simulink model "Benchmark_IEEE_standardn4"  (R2018a)
settings: Solver=ode45  StartTime=0.0  StopTime=200  FixedStep=1e-4  RelTol=1e-5  EnableMultiTasking=on
undefined symbols (not defined in the file): a, Aex, b, Bex, D, delta0, dVref, Ed_dash0, Edc_dash0, Efd0, Efdmax, Efdmax_dc, Efdmin, Efdmin_dc, Eq_dash0, j, Ka, KA, Kad, kc, Kd, Ke, Kf, Ki, Kp, Ks, M, MM, P18cor2, P50cor2, Psi1d0, Psi2q0, Sm0, T11, T12, T21, T22, T31, T32, Ta, Tc, Td, Td0d, Td0dd, Te, Tf, theta, Tm0, Tq0d, Tq0dd, Tr, Tw, V, v1, V18cor, V2, V50cor, V_Ka0, V_Ki0, Vg ... (+15)
settings Model: Creator=aks11  LastModifiedBy=sanam
settings DataIOCC: SaveFormat=StructureWithTime  SignalLoggingSaveFormat=ModelDataLogs  SaveOutput=off  SaveState=on  SignalLogging=off  DSMLogging=off
settings OptimizationCC: BlockReduction=off  DefaultParameterBehavior=Inlined  BufferReuse=off  ExpressionDepthLimit=2147483647  LifeSpan=inf  SimCompilerOptimization=on
settings DebuggingCC: AlgebraicLoopMsg=none  UnderspecifiedInitializationDetection=Classic  MergeDetectMultiDrivingBlocksExec=none  FcnCallInpInsideContextMsg=warning  UnconnectedInputMsg=none  UnconnectedOutputMsg=none  UnconnectedLineMsg=none  StateNameClashWarn=warning  SFUnexpectedBacktrackingDiag=warning  SFNoUnconditionalDefaultTransitionDiag=warning  SFExecutionAtInitializationDiag=none
settings HardwareCC: ProdBitPerPointer=32  ProdBitPerSizeT=32  ProdBitPerPtrDiffT=32  ProdLargestAtomicFloat=None  ProdIntDivRoundTo=Undefined  ProdEndianess=Unspecified  ProdWordSize=32  ProdHWDeviceType=32-bit Generic
settings ModelReferenceCC: PropagateSignalLabelsOutOfModel=off
settings CodeAppCC: StateflowObjectComments=on
settings GRTTargetCC: TargetLangStandard=C89/C90 (ANSI)  GeneratePreprocessorConditionals=Disable all  CombineOutputUpdateFcns=off  GRTInterface=on
settings ConfigComp: CovMetricSettings=dw  CovHtmlReporting=on  CovSaveCumulativeToWorkspaceVar=on  CovSaveSingleToWorkspaceVar=on  CovExternalEMLEnable=off

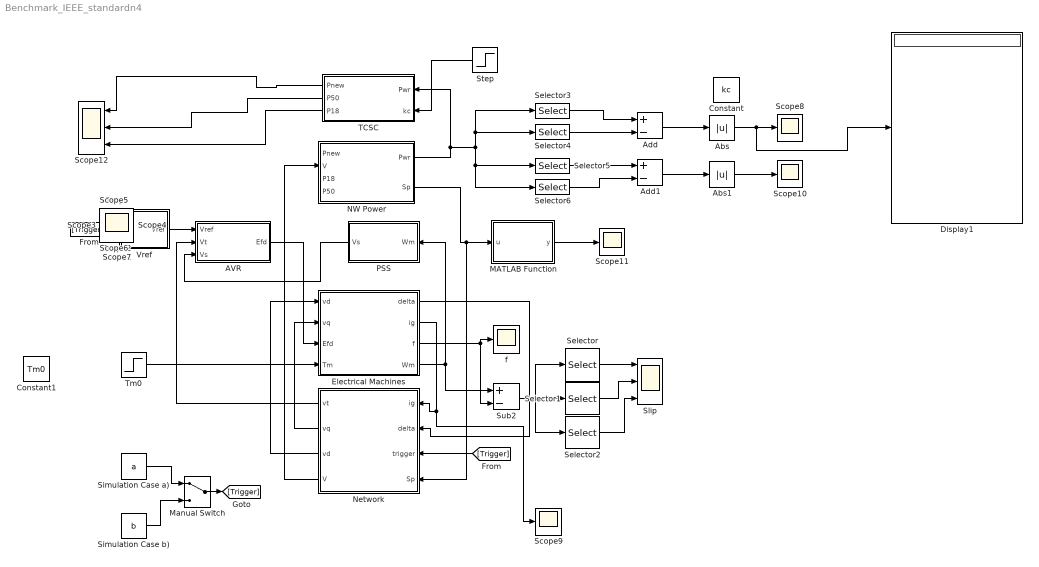
== system Benchmark_IEEE_standardn4 ==
  AVR : Subsystem
  Abs : Abs
  Abs1 : Abs
  Add : Sum  Inputs=+-
  Add1 : Sum  Inputs=+-
  Constant : Constant  Value=kc
  Constant1 : Constant  Value=Tm0
  Display1 : Display
  Electrical Machines : Subsystem
  MATLAB Function : MATLAB Function  TreatAsAtomicUnit=on
  Manual Switch : ManualSwitch
  NW Power : Subsystem
  Network : Subsystem
  PSS : Subsystem
  Scope{,1..11} (12 alike) : Scope
  Scope12 : Scope  NumInputPorts=3
  Selector : Selector  IndexOptions=Index vector (dialog)  Indices=4  OutputSizes=1
  Selector1 : Selector  IndexOptions=Index vector (dialog)  Indices=9  OutputSizes=1
  Selector2 : Selector  IndexOptions=Index vector (dialog)  Indices=15  OutputSizes=1
  Selector3 : Selector  IndexOptions=Index vector (dialog)  Indices=13  OutputSizes=1
  Selector4 : Selector  IndexOptions=Index vector (dialog)  Indices=17  OutputSizes=1
  Selector5 : Selector  IndexOptions=Index vector (dialog)  Indices=16  OutputSizes=1
  Selector6 : Selector  IndexOptions=Index vector (dialog)  Indices=18  OutputSizes=1
  Simulation Case a) : Constant  Value=a
  Simulation Case b) : Constant  Value=b
  Slip : Scope  NumInputPorts=3
  Step : Step  Time=0  After=0.5  SampleTime=0
  Sub2 : Sum  Inputs=+-
  TCSC : Subsystem
  Tm0 : Step  Time=0  Before=Tm0  After=Tm0  SampleTime=0
  Vref : Subsystem
  f : Scope
  wires:
  Electrical Machines/2(ig) -> Scope9/1, Network/1(ig)
  Network/1(vt) -> AVR/2(Vt)
  Network/2(vq) -> Electrical Machines/2(vq)
  Network/3(vd) -> Electrical Machines/1(vd)
  Tm0/1 -> Electrical Machines/4(Tm)
  PSS/1(Vs) -> AVR/3(Vs)
  AVR/1(Efd) -> Electrical Machines/3("Efd ")
  Selector/1 -> Slip/1
  Electrical Machines/3(f) -> f/1, Sub2/2
  Electrical Machines/4(Wm) -> Sub2/1, PSS/1(Wm)
  Electrical Machines/1(delta) -> Network/2(delta)
  Sub2/1 -> Selector2/1, Selector/1, Selector1/1
  Vref/1(Vref) -> AVR/1(Vref)
  Simulation Case a)/1 -> Manual Switch/1
  Simulation Case b)/1 -> Manual Switch/2
  Manual Switch/1 -> [Trigger]
  [Trigger] -> Vref/1(trigger)
  [Trigger] -> Network/3(trigger)
  Selector1/1 -> Slip/2
  Selector2/1 -> Slip/3
  NW Power/1(Pwr) -> Selector3/1, Selector4/1, Selector6/1, Selector5/1, TCSC/1(Pwr)
  TCSC/1(Pnew) -> Scope12/1
  TCSC/2(P50) -> Scope12/2
  TCSC/3(P18) -> Scope12/3
  Selector3/1 -> Add/1
  Selector4/1 -> Add/2
  Selector5/1 -> Add1/1
  Selector6/1 -> Add1/2
  Add/1 -> Abs/1
  Add1/1 -> Abs1/1
  Abs/1 -> Display1/1, Scope8/1
  Abs1/1 -> Scope10/1
  NW Power/2(Sp) -> Network/4(Sp), MATLAB Function/1(u)
  MATLAB Function/1(y) -> Scope11/1
  Network/4(V) -> NW Power/2(V)
  Step/1 -> TCSC/2(kc)

== system Benchmark_IEEE_standardn4/AVR ==
  Vref : Inport
  Vt : Inport  Port=2
  Vs : Inport  Port=3
  AVR (DC4B) : Subsystem
  AVR (ST1A) : Subsystem
  Manual : Subsystem
  Sum7 : Sum  Inputs=+++
  Efd : Outport
  wires:
  Sum7/1 -> Efd/1
  AVR (DC4B)/1(Efd) -> Sum7/2
  AVR (ST1A)/1(Efd) -> Sum7/1
  Vref/1 -> Manual/1(Vref), AVR (DC4B)/1(Vref), AVR (ST1A)/1(Vref)
  Vt/1 -> AVR (DC4B)/2(Vt), AVR (ST1A)/2(Vt)
  Vs/1 -> AVR (DC4B)/3(Vs), AVR (ST1A)/3(Vs)
  Manual/1(Efd3) -> Sum7/3

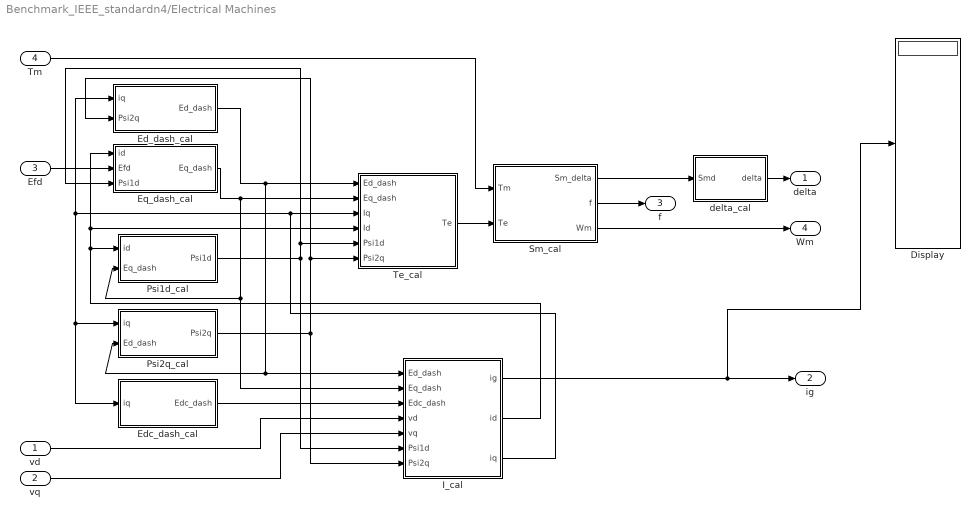
== system Benchmark_IEEE_standardn4/Electrical Machines ==
  vd : Inport
  vq : Inport  Port=2
  "Efd " : Inport  Port=3
  Tm : Inport  Port=4
  Display : Display
  Ed_dash_cal : Subsystem
  Edc_dash_cal : Subsystem
  Eq_dash_cal : Subsystem
  I_cal : Subsystem
  Psi1d_cal : Subsystem
  Psi2q_cal : Subsystem
  Sm_cal : Subsystem
  Te_cal : Subsystem
  delta_cal : Subsystem
  delta : Outport
  ig : Outport  Port=2
  f : Outport  Port=3
  Wm : Outport  Port=4
  wires:
  Ed_dash_cal/1(Ed_dash) -> Te_cal/1(Ed_dash), I_cal/1(Ed_dash), Psi2q_cal/2(Ed_dash)
  Eq_dash_cal/1(Eq_dash) -> Te_cal/2(Eq_dash), I_cal/2(Eq_dash), Psi1d_cal/2(Eq_dash)
  "Efd "/1 -> Eq_dash_cal/2(Efd)
  Edc_dash_cal/1(Edc_dash) -> I_cal/3(Edc_dash)
  vd/1 -> I_cal/4(vd)
  vq/1 -> I_cal/5(vq)
  I_cal/3(iq) -> Te_cal/3(Iq), Ed_dash_cal/1(iq), Edc_dash_cal/1(iq), Psi2q_cal/1(iq)
  I_cal/1(ig) -> Display/1, ig/1
  I_cal/2(id) -> Eq_dash_cal/1(id), Te_cal/4(Id), Psi1d_cal/1(id)
  Psi2q_cal/1(Psi2q) -> Te_cal/6(Psi2q), Ed_dash_cal/2(Psi2q), I_cal/7(Psi2q)
  Psi1d_cal/1(Psi1d) -> Te_cal/5(Psi1d), Eq_dash_cal/3(Psi1d), I_cal/6(Psi1d)
  Sm_cal/2(f) -> f/1
  Sm_cal/1(Sm_delta) -> delta_cal/1(Smd)
  delta_cal/1(delta) -> delta/1
  Sm_cal/3(Wm) -> Wm/1
  Te_cal/1(Te) -> Sm_cal/2(Te)
  Tm/1 -> Sm_cal/1(Tm)

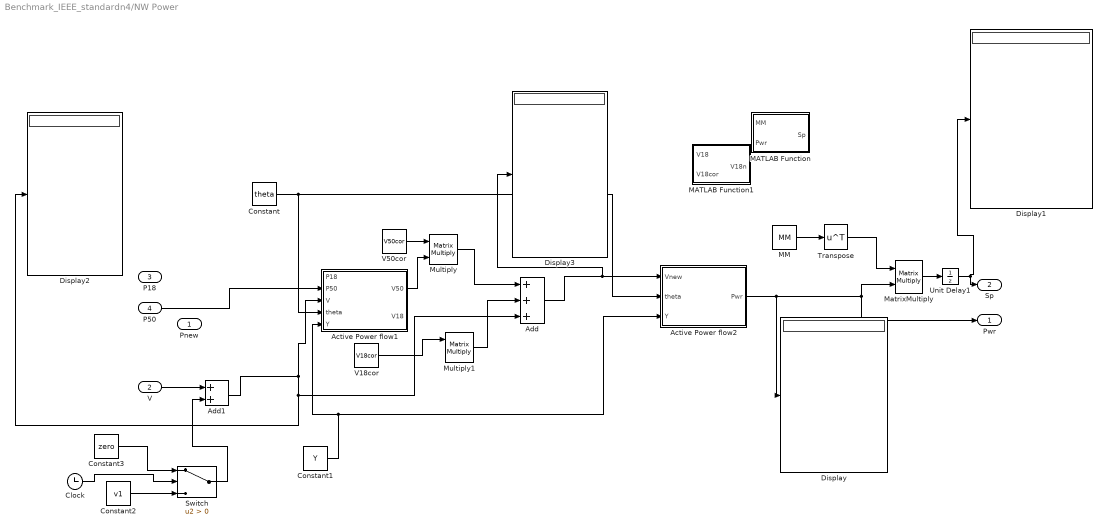
== system Benchmark_IEEE_standardn4/NW Power ==
  Pnew : Inport
  V : Inport  Port=2
  P18 : Inport  Port=3
  P50 : Inport  Port=4
  Active Power flow1 : MATLAB Function  TreatAsAtomicUnit=on
  Active Power flow2 : MATLAB Function  TreatAsAtomicUnit=on
  Add : Sum  Inputs=3
  Add1 : Sum
  Clock : Clock
  Constant : Constant  Value=theta
  Constant1 : Constant  Value=Y
  Constant2 : Constant  Value=v1
  Constant3 : Constant  Value=zero
  Display{,1..3} (4 alike) : Display
  MATLAB Function : MATLAB Function  TreatAsAtomicUnit=on
  MATLAB Function1 : MATLAB Function  TreatAsAtomicUnit=on
  MM : Constant  Value=MM
  MatrixMultiply : Product  Multiplication=Matrix(*)
  Multiply : Product  Multiplication=Matrix(*)
  Multiply1 : Product  Multiplication=Matrix(*)
  Switch : Switch  Criteria=u2 > Threshold
  Transpose : Math  Operator=transpose  SaturateOnIntegerOverflow=on
  Unit Delay1 : UnitDelay  SampleTime=-1
  V18cor : Constant  Value=V18cor
  V50cor : Constant  Value=V50cor
  Pwr : Outport
  Sp : Outport  Port=2
  wires:
  Constant1/1 -> Active Power flow1/5(Y), Active Power flow2/3(Y)
  Constant/1 -> Active Power flow1/4(theta), Active Power flow2/2(theta)
  V50cor/1 -> Multiply/1
  Active Power flow1/1(V50) -> Multiply/2
  Multiply/1 -> Add/1
  Active Power flow2/1(Pwr) -> Display/1, MatrixMultiply/2, Pwr/1
  MM/1 -> Transpose/1
  Multiply1/1 -> Add/2
  Unit Delay1/1 -> Display1/1, Sp/1
  MatrixMultiply/1 -> Unit Delay1/1
  V18cor/1 -> Multiply1/1
  Add/1 -> Display3/1, Active Power flow2/1(Vnew)
  Transpose/1 -> MatrixMultiply/1
  Add1/1 -> Display2/1, Add/3, Active Power flow1/3(V)
  V/1 -> Add1/1
  Constant2/1 -> Switch/3
  Clock/1 -> Switch/2
  Constant3/1 -> Switch/1
  Switch/1 -> Add1/2
  P50/1 -> Active Power flow1/2(P50)

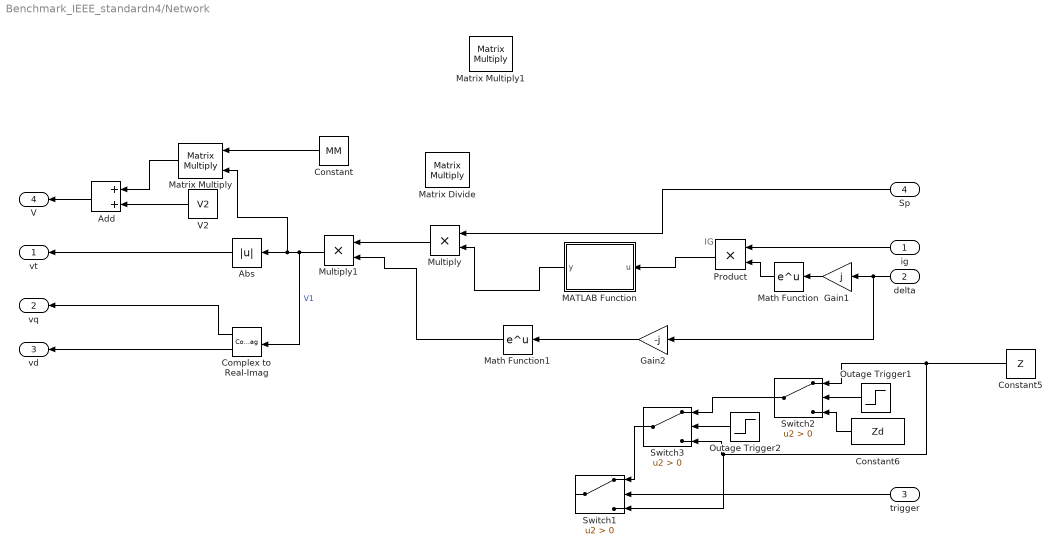
== system Benchmark_IEEE_standardn4/Network ==
  note: IG
  ig : Inport
  delta : Inport  Port=2
  trigger : Inport  Port=3
  Sp : Inport  Port=4
  Abs : Abs
  Add : Sum
  Complex to Real-Imag : ComplexToRealImag
  Constant : Constant  Value=MM
  Constant5 : Constant  Value=Z
  Constant6 : Constant  Value=Zd
  Gain1 : Gain  Gain=j
  Gain2 : Gain  Gain=-j
  MATLAB Function : MATLAB Function  TreatAsAtomicUnit=on
  Math Function : Math  SaturateOnIntegerOverflow=on
  Math Function1 : Math  SaturateOnIntegerOverflow=on
  Matrix Divide : Product  Inputs=**  Multiplication=Matrix(*)
  Matrix Multiply : Product  Multiplication=Matrix(*)
  Matrix Multiply1 : Product  Multiplication=Matrix(*)
  Multiply : Product
  Multiply1 : Product
  Outage Trigger1 : Step  Before=1  After=0  SampleTime=0
  Outage Trigger2 : Step  Time=11  Before=1  After=0  SampleTime=0
  Product : Product  RndMeth=Zero
  Switch1 : Switch  Criteria=u2 > Threshold
  Switch2 : Switch  Criteria=u2 > Threshold
  Switch3 : Switch  Criteria=u2 > Threshold
  V2 : Constant  Value=V2
  vt : Outport
  vq : Outport  Port=2
  vd : Outport  Port=3
  V : Outport  Port=4
  wires:
  Math Function/1 -> Product/2
  Math Function1/1 -> Multiply1/2
  Gain2/1 -> Math Function1/1
  Gain1/1 -> Math Function/1
  Abs/1 -> vt/1
  Complex to Real-Imag/1 -> vq/1
  ig/1 -> Product/1
  Multiply1/1 -> Complex to Real-Imag/1, Matrix Multiply/2, Abs/1  "V1"
  Multiply/1 -> Multiply1/1
  delta/1 -> Gain2/1, Gain1/1
  Outage Trigger1/1 -> Switch2/2
  Constant6/1 -> Switch2/3
  Complex to Real-Imag/2 -> vd/1
  Outage Trigger2/1 -> Switch3/2
  Switch2/1 -> Switch3/1
  Switch3/1 -> Switch1/1
  trigger/1 -> Switch1/2
  Constant5/1 -> Switch1/3, Switch3/3, Switch2/1
  Product/1 -> MATLAB Function/1(u)
  Sp/1 -> Multiply/1
  Constant/1 -> Matrix Multiply/1
  Matrix Multiply/1 -> Add/1
  V2/1 -> Add/2
  Add/1 -> V/1
  MATLAB Function/1(y) -> Multiply/2

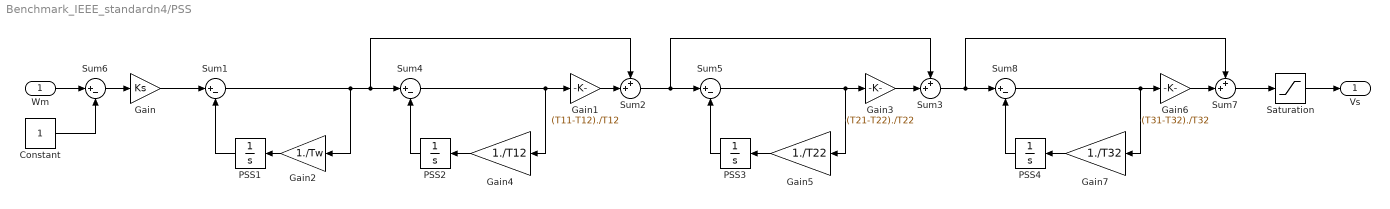
== system Benchmark_IEEE_standardn4/PSS ==
  Wm : Inport
  Constant : Constant
  Gain : Gain  Gain=Ks
  Gain1 : Gain  Gain=(T11-T12)./T12
  Gain2 : Gain  Gain=1./Tw
  Gain3 : Gain  Gain=(T21-T22)./T22
  Gain4 : Gain  Gain=1./T12
  Gain5 : Gain  Gain=1./T22
  Gain6 : Gain  Gain=(T31-T32)./T32
  Gain7 : Gain  Gain=1./T32
  PSS{1..4} (4 alike) : Integrator  UpperSaturationLimit=Efdmax  LowerSaturationLimit=Efdmin
  Saturation : Saturate  UpperLimit=Vs_max  LowerLimit=Vs_min
  Sum{1,4..6,8} (5 alike) : Sum  Inputs=|+-
  Sum2 : Sum  Inputs=++|
  Sum3 : Sum  Inputs=++|
  Sum7 : Sum  Inputs=++|
  Vs : Outport
  wires:
  Gain/1 -> Sum1/1
  Saturation/1 -> Vs/1
  Sum1/1 -> Gain2/1, Sum4/1, Sum2/1
  PSS1/1 -> Sum1/2
  Gain2/1 -> PSS1/1
  Sum4/1 -> Gain4/1, Gain1/1
  PSS2/1 -> Sum4/2
  Gain4/1 -> PSS2/1
  Gain1/1 -> Sum2/2
  Sum2/1 -> Sum3/1, Sum5/1
  Sum5/1 -> Gain3/1, Gain5/1
  PSS3/1 -> Sum5/2
  Gain5/1 -> PSS3/1
  Gain3/1 -> Sum3/2
  Wm/1 -> Sum6/1
  Sum6/1 -> Gain/1
  Constant/1 -> Sum6/2
  Sum7/1 -> Saturation/1
  Sum3/1 -> Sum7/1, Sum8/1
  Sum8/1 -> Gain6/1, Gain7/1
  PSS4/1 -> Sum8/2
  Gain7/1 -> PSS4/1
  Gain6/1 -> Sum7/2

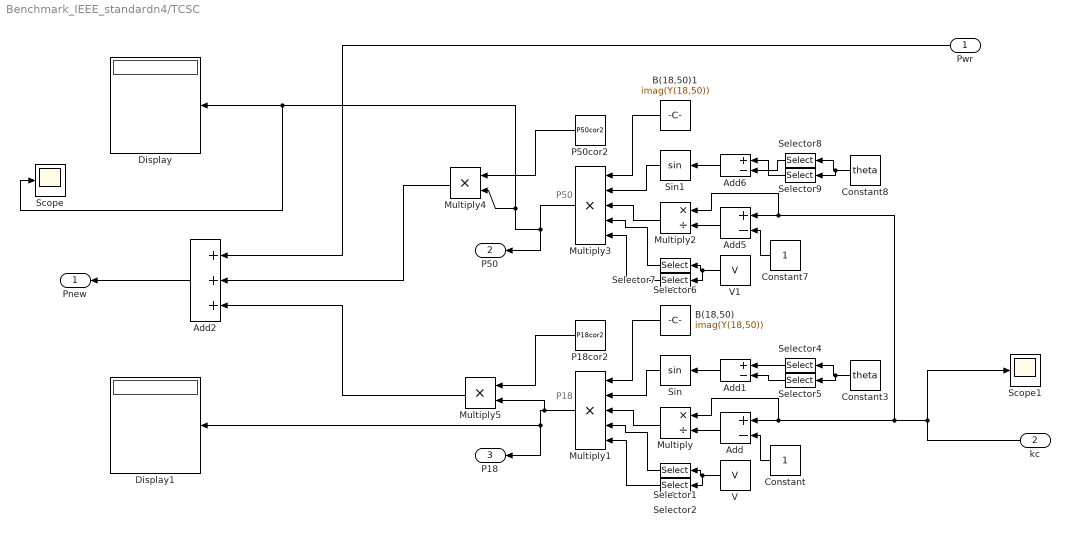
== system Benchmark_IEEE_standardn4/TCSC ==
  note: P18
  note: P50
  Pwr : Inport
  kc : Inport  Port=2
  Add{,1,5..6} (4 alike) : Sum  Inputs=+-
  Add2 : Sum  Inputs=3
  B(18,50) : Constant  Value=imag(Y(18,50))
  B(18,50)1 : Constant  Value=imag(Y(18,50))
  Constant : Constant
  Constant3 : Constant  Value=theta
  Constant7 : Constant
  Constant8 : Constant  Value=theta
  Display : Display
  Display1 : Display
  Multiply : Product  Inputs=*/
  Multiply1 : Product  Inputs=*****
  Multiply2 : Product  Inputs=*/
  Multiply3 : Product  Inputs=*****
  Multiply4 : Product
  Multiply5 : Product
  P18cor2 : Constant  Value=P18cor2
  P50cor2 : Constant  Value=P50cor2
  Scope : Scope
  Scope1 : Scope
  Selector{1,4,6,8} (4 alike) : Selector  IndexOptions=Index vector (dialog)  Indices=18  OutputSizes=1
  Selector{2,5,7,9} (4 alike) : Selector  IndexOptions=Index vector (dialog)  Indices=50  OutputSizes=1
  Sin : Trigonometry
  Sin1 : Trigonometry
  V : Constant  Value=V
  V1 : Constant  Value=V
  Pnew : Outport
  P50 : Outport  Port=2
  P18 : Outport  Port=3
  wires:
  Sin/1 -> Multiply1/2
  B(18,50)/1 -> Multiply1/1
  Multiply2/1 -> Multiply3/3
  Constant7/1 -> Add5/2
  V/1 -> Selector2/1, Selector1/1
  Sin1/1 -> Multiply3/2
  kc/1 -> Scope1/1, Multiply2/1, Add5/1, Multiply/1, Add/1
  Selector2/1 -> Multiply1/5
  V1/1 -> Selector7/1, Selector6/1
  Add/1 -> Multiply/2
  B(18,50)1/1 -> Multiply3/1
  Multiply/1 -> Multiply1/3
  Constant/1 -> Add/2
  Selector7/1 -> Multiply3/5
  Constant8/1 -> Selector9/1, Selector8/1
  Selector6/1 -> Multiply3/4
  Constant3/1 -> Selector5/1, Selector4/1
  Add6/1 -> Sin1/1
  Selector1/1 -> Multiply1/4
  Add1/1 -> Sin/1
  Selector4/1 -> Add1/1
  Selector5/1 -> Add1/2
  Add5/1 -> Multiply2/2
  Selector9/1 -> Add6/1
  Selector8/1 -> Add6/2
  P50cor2/1 -> Multiply4/1
  P18cor2/1 -> Multiply5/1
  Pwr/1 -> Add2/1
  Multiply4/1 -> Add2/2
  Multiply5/1 -> Add2/3
  Multiply1/1 -> Multiply5/2, Display1/1, P18/1
  Multiply3/1 -> Multiply4/2, Scope/1, Display/1, P50/1
  Add2/1 -> Pnew/1

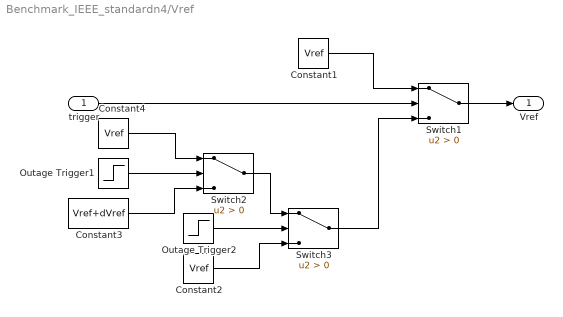
== system Benchmark_IEEE_standardn4/Vref ==
  trigger : Inport
  Constant1 : Constant  Value=Vref
  Constant2 : Constant  Value=Vref
  Constant3 : Constant  Value=Vref+dVref
  Constant4 : Constant  Value=Vref
  Outage Trigger1 : Step  Before=1  After=0  SampleTime=0
  Outage Trigger2 : Step  Time=11  Before=1  After=0  SampleTime=0
  Switch1 : Switch  Criteria=u2 > Threshold
  Switch2 : Switch  Criteria=u2 > Threshold
  Switch3 : Switch  Criteria=u2 > Threshold
  Vref : Outport
  wires:
  Constant1/1 -> Switch1/1
  Constant2/1 -> Switch3/3
  Outage Trigger2/1 -> Switch3/2
  Switch3/1 -> Switch1/3
  Switch1/1 -> Vref/1
  Constant3/1 -> Switch2/3
  Outage Trigger1/1 -> Switch2/2
  Switch2/1 -> Switch3/1
  Constant4/1 -> Switch2/1
  trigger/1 -> Switch1/2

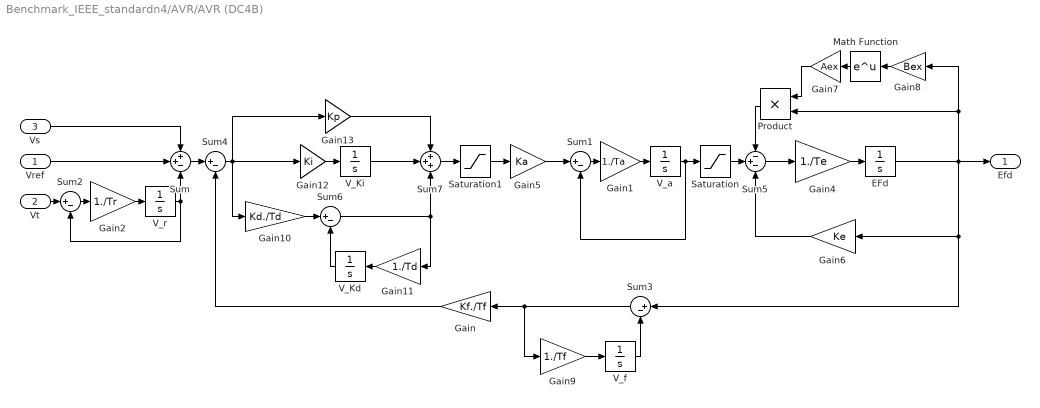
== system Benchmark_IEEE_standardn4/AVR/AVR (DC4B) ==
  Vref : Inport
  Vt : Inport  Port=2
  Vs : Inport  Port=3
  EFd : Integrator  InitialCondition=Efd0.*Kad  UpperSaturationLimit=Efdmax_dc  LowerSaturationLimit=Efdmin_dc
  Gain : Gain  Gain=Kf./Tf
  Gain1 : Gain  Gain=1./Ta
  Gain10 : Gain  Gain=Kd./Td
  Gain11 : Gain  Gain=1./Td
  Gain12 : Gain  Gain=Ki
  Gain13 : Gain  Gain=Kp
  Gain2 : Gain  Gain=1./Tr
  Gain4 : Gain  Gain=1./Te
  Gain5 : Gain  Gain=Ka
  Gain6 : Gain  Gain=Ke
  Gain7 : Gain  Gain=Aex
  Gain8 : Gain  Gain=Bex
  Gain9 : Gain  Gain=1./Tf
  Math Function : Math  SaturateOnIntegerOverflow=on
  Product : Product  RndMeth=Zero
  Saturation : Saturate  UpperLimit=Efdmax_dc  LowerLimit=Efdmin_dc
  Saturation1 : Saturate  UpperLimit=Efdmax_dc./Ka  LowerLimit=Efdmin_dc./Ka
  Sum : Sum  Inputs=++-
  Sum{1..4,6} (5 alike) : Sum  Inputs=|+-
  Sum5 : Sum  Inputs=-+-
  Sum7 : Sum  Inputs=+++
  V_Kd : Integrator  UpperSaturationLimit=Efdmax  LowerSaturationLimit=Efdmin
  V_Ki : Integrator  InitialCondition=V_Ki0  UpperSaturationLimit=Efdmax_dc  LowerSaturationLimit=Efdmin_dc
  V_a : Integrator  InitialCondition=V_Ka0  UpperSaturationLimit=Efdmax  LowerSaturationLimit=Efdmin
  V_f : Integrator  InitialCondition=Efd0.*Kad  UpperSaturationLimit=Efdmax  LowerSaturationLimit=Efdmin
  V_r : Integrator  InitialCondition=Vg  UpperSaturationLimit=Efdmax  LowerSaturationLimit=Efdmin
  Efd : Outport
  wires:
  Gain8/1 -> Math Function/1
  Math Function/1 -> Gain7/1
  Sum1/1 -> Gain1/1
  Gain1/1 -> V_a/1
  V_a/1 -> Sum1/2, Saturation/1
  Gain5/1 -> Sum1/1
  Sum5/1 -> Gain4/1
  Gain4/1 -> EFd/1
  Sum2/1 -> Gain2/1
  Gain2/1 -> V_r/1
  V_r/1 -> Sum2/2, Sum/3
  Vref/1 -> Sum/2
  Vt/1 -> Sum2/1
  Product/1 -> Sum5/1
  Gain6/1 -> Sum5/3
  Gain7/1 -> Product/1
  Saturation/1 -> Sum5/2
  EFd/1 -> Product/2, Gain8/1, Efd/1, Sum3/1, Gain6/1
  Gain9/1 -> V_f/1
  Sum3/1 -> Gain/1, Gain9/1
  Sum/1 -> Sum4/1
  V_Kd/1 -> Sum6/2
  Gain11/1 -> V_Kd/1
  Gain10/1 -> Sum6/1
  Sum6/1 -> Sum7/3, Gain11/1
  Gain12/1 -> V_Ki/1
  V_Ki/1 -> Sum7/2
  Gain13/1 -> Sum7/1
  Sum7/1 -> Saturation1/1
  Sum4/1 -> Gain13/1, Gain12/1, Gain10/1
  Saturation1/1 -> Gain5/1
  Vs/1 -> Sum/1
  V_f/1 -> Sum3/2
  Gain/1 -> Sum4/2

== system Benchmark_IEEE_standardn4/AVR/AVR (ST1A) ==
  Vref : Inport
  Vt : Inport  Port=2
  Vs : Inport  Port=3
  EFdd2 : Integrator  InitialCondition=Vg  UpperSaturationLimit=Efdmax  LowerSaturationLimit=Efdmin
  Gain2 : Gain  Gain=1./Tr
  Gain5 : Gain  Gain=KA
  Saturation : Saturate  UpperLimit=Efdmax  LowerLimit=Efdmin
  Sum : Sum  Inputs=++-
  Sum2 : Sum  Inputs=|+-
  Efd : Outport
  wires:
  Saturation/1 -> Efd/1
  Gain5/1 -> Saturation/1
  Sum2/1 -> Gain2/1
  Gain2/1 -> EFdd2/1
  EFdd2/1 -> Sum2/2, Sum/3
  Vref/1 -> Sum/2
  Vs/1 -> Sum/1
  Vt/1 -> Sum2/1
  Sum/1 -> Gain5/1

== system Benchmark_IEEE_standardn4/AVR/Manual ==
  Vref : Inport
  Gain9 : Gain  Gain=Vref_Manual
  Efd3 : Outport
  wires:
  Vref/1 -> Gain9/1
  Gain9/1 -> Efd3/1

== system Benchmark_IEEE_standardn4/Electrical Machines/Ed_dash_cal ==
  iq : Inport
  Psi2q : Inport  Port=2
  Add2 : Sum  Inputs=+-
  Add3 : Sum  Inputs=-+
  Add4 : Sum  Inputs=-+-
  Edd : Integrator  InitialCondition=Ed_dash0
  Gain : Gain  Gain=1./Tq0d
  Gain1 : Gain  Gain=xq-xqd
  Gain2 : Gain  Gain=xqd-xls
  Gain3 : Gain  Gain=(xqd-xqdd)./((xqd-xls).^2)
  Ed_dash : Outport
  wires:
  Gain3/1 -> Add3/2
  Add4/1 -> Gain3/1
  Gain2/1 -> Add4/2
  Psi2q/1 -> Add4/1
  iq/1 -> Gain2/1, Add3/1
  Add3/1 -> Gain1/1
  Edd/1 -> Add4/3, Add2/2, Ed_dash/1  "Ed_dash"
  Gain/1 -> Edd/1
  Add2/1 -> Gain/1
  Gain1/1 -> Add2/1

== system Benchmark_IEEE_standardn4/Electrical Machines/Edc_dash_cal ==
  iq : Inport
  Add2 : Sum  Inputs=+-
  Edcd : Integrator  InitialCondition=Edc_dash0
  Gain : Gain  Gain=1./Tc
  Gain1 : Gain  Gain=xddd-xqdd
  Edc_dash : Outport
  wires:
  Gain1/1 -> Add2/1
  Add2/1 -> Gain/1
  Gain/1 -> Edcd/1
  Edcd/1 -> Add2/2, Edc_dash/1  "Edc_dash"
  iq/1 -> Gain1/1

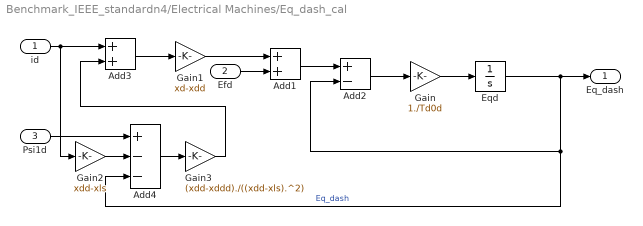
== system Benchmark_IEEE_standardn4/Electrical Machines/Eq_dash_cal ==
  id : Inport
  Efd : Inport  Port=2
  Psi1d : Inport  Port=3
  Add1 : Sum
  Add2 : Sum  Inputs=+-
  Add3 : Sum
  Add4 : Sum  Inputs=+--
  Eqd : Integrator  InitialCondition=Eq_dash0
  Gain : Gain  Gain=1./Td0d
  Gain1 : Gain  Gain=xd-xdd
  Gain2 : Gain  Gain=xdd-xls
  Gain3 : Gain  Gain=(xdd-xddd)./((xdd-xls).^2)
  Eq_dash : Outport
  wires:
  Gain1/1 -> Add1/1
  Efd/1 -> Add1/2
  Add1/1 -> Add2/1
  Add2/1 -> Gain/1
  Gain/1 -> Eqd/1
  Eqd/1 -> Eq_dash/1, Add2/2, Add4/3  "Eq_dash"
  Add3/1 -> Gain1/1
  id/1 -> Add3/1, Gain2/1
  Psi1d/1 -> Add4/1
  Gain2/1 -> Add4/2
  Add4/1 -> Gain3/1
  Gain3/1 -> Add3/2

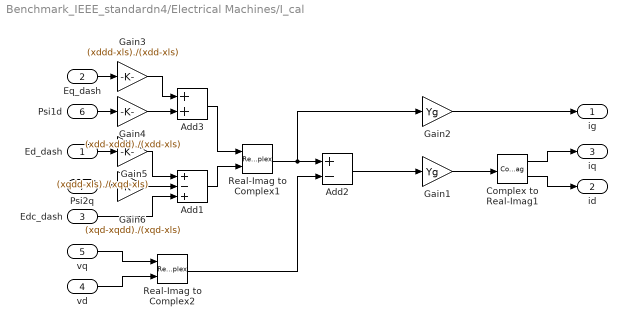
== system Benchmark_IEEE_standardn4/Electrical Machines/I_cal ==
  Ed_dash : Inport
  Eq_dash : Inport  Port=2
  Edc_dash : Inport  Port=3
  vd : Inport  Port=4
  vq : Inport  Port=5
  Psi1d : Inport  Port=6
  Psi2q : Inport  Port=7
  Add1 : Sum  Inputs=+-+
  Add2 : Sum  Inputs=+-
  Add3 : Sum
  Complex to Real-Imag1 : ComplexToRealImag
  Gain1 : Gain  Gain=Yg
  Gain2 : Gain  Gain=Yg
  Gain3 : Gain  Gain=(xddd-xls)./(xdd-xls)
  Gain4 : Gain  Gain=(xdd-xddd)./(xdd-xls)
  Gain5 : Gain  Gain=(xqdd-xls)./(xqd-xls)
  Gain6 : Gain  Gain=(xqd-xqdd)./(xqd-xls)
  Real-Imag to Complex1 : RealImagToComplex
  Real-Imag to Complex2 : RealImagToComplex
  ig : Outport
  id : Outport  Port=2
  iq : Outport  Port=3
  wires:
  Ed_dash/1 -> Gain5/1
  Add1/1 -> Real-Imag to Complex1/2
  vq/1 -> Real-Imag to Complex2/1
  vd/1 -> Real-Imag to Complex2/2
  Real-Imag to Complex1/1 -> Add2/1, Gain2/1
  Add2/1 -> Gain1/1
  Real-Imag to Complex2/1 -> Add2/2
  Gain2/1 -> ig/1
  Complex to Real-Imag1/2 -> id/1
  Complex to Real-Imag1/1 -> iq/1
  Gain1/1 -> Complex to Real-Imag1/1
  Eq_dash/1 -> Gain3/1
  Gain3/1 -> Add3/1
  Psi1d/1 -> Gain4/1
  Gain4/1 -> Add3/2
  Add3/1 -> Real-Imag to Complex1/1
  Edc_dash/1 -> Add1/3
  Gain5/1 -> Add1/1
  Psi2q/1 -> Gain6/1
  Gain6/1 -> Add1/2

== system Benchmark_IEEE_standardn4/Electrical Machines/Psi1d_cal ==
  id : Inport
  Eq_dash : Inport  Port=2
  Add2 : Sum  Inputs=++-
  Gain : Gain  Gain=1./Td0dd
  Gain1 : Gain  Gain=xdd-xls
  Psi_1d : Integrator  InitialCondition=Psi1d0
  Psi1d : Outport
  wires:
  id/1 -> Gain1/1
  Psi_1d/1 -> Psi1d/1, Add2/3  "Phi1d"
  Gain/1 -> Psi_1d/1
  Add2/1 -> Gain/1
  Gain1/1 -> Add2/1
  Eq_dash/1 -> Add2/2

== system Benchmark_IEEE_standardn4/Electrical Machines/Psi2q_cal ==
  iq : Inport
  Ed_dash : Inport  Port=2
  Add2 : Sum  Inputs=+--
  Gain : Gain  Gain=1./Tq0dd
  Gain1 : Gain  Gain=xqd-xls
  Psi_2q : Integrator  InitialCondition=Psi2q0
  Psi2q : Outport
  wires:
  Ed_dash/1 -> Add2/2
  Gain1/1 -> Add2/1
  Add2/1 -> Gain/1
  Gain/1 -> Psi_2q/1
  Psi_2q/1 -> Add2/3, Psi2q/1  "Psi2q"
  iq/1 -> Gain1/1

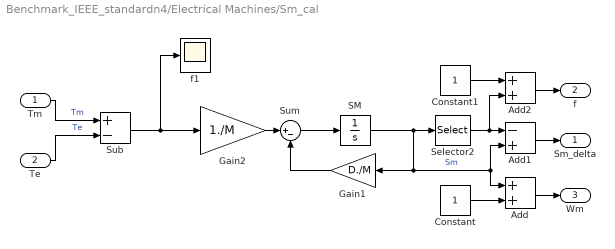
== system Benchmark_IEEE_standardn4/Electrical Machines/Sm_cal ==
  Tm : Inport
  Te : Inport  Port=2
  Add : Sum
  Add1 : Sum  Inputs=-+
  Add2 : Sum
  Constant : Constant
  Constant1 : Constant
  Gain1 : Gain  Gain=D./M
  Gain2 : Gain  Gain=1./M
  SM : Integrator  InitialCondition=Sm0
  Selector2 : Selector  IndexOptions=Index vector (dialog)  Indices=swing_index  OutputSizes=1
  Sub : Sum  Inputs=+-
  Sum : Sum  Inputs=|+-
  f1 : Scope
  Sm_delta : Outport
  f : Outport  Port=2
  Wm : Outport  Port=3
  wires:
  Tm/1 -> Sub/1  "Tm"
  Te/1 -> Sub/2  "Te"
  Gain1/1 -> Sum/2
  Gain2/1 -> Sum/1
  SM/1 -> Gain1/1, Add/1, Add1/2, Selector2/1  "Sm"
  Selector2/1 -> Add2/2, Add1/1
  Add1/1 -> Sm_delta/1
  Constant/1 -> Add/2
  Add/1 -> Wm/1
  Constant1/1 -> Add2/1
  Add2/1 -> f/1
  Sum/1 -> SM/1
  Sub/1 -> Gain2/1, f1/1

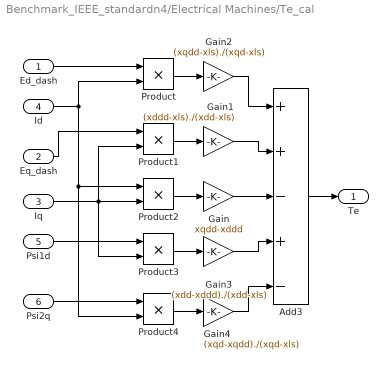
== system Benchmark_IEEE_standardn4/Electrical Machines/Te_cal ==
  Ed_dash : Inport
  Eq_dash : Inport  Port=2
  Iq : Inport  Port=3
  Id : Inport  Port=4
  Psi1d : Inport  Port=5
  Psi2q : Inport  Port=6
  Add3 : Sum  Inputs=++-+-
  Gain : Gain  Gain=xqdd-xddd
  Gain1 : Gain  Gain=(xddd-xls)./(xdd-xls)
  Gain2 : Gain  Gain=(xqdd-xls)./(xqd-xls)
  Gain3 : Gain  Gain=(xdd-xddd)./(xdd-xls)
  Gain4 : Gain  Gain=(xqd-xqdd)./(xqd-xls)
  Product{,1..4} (5 alike) : Product  RndMeth=Zero
  Te : Outport
  wires:
  Add3/1 -> Te/1
  Eq_dash/1 -> Product1/1
  Id/1 -> Product/2, Product2/1, Product4/2
  Ed_dash/1 -> Product/1
  Iq/1 -> Product2/2, Product3/2, Product1/2
  Product2/1 -> Gain/1
  Product1/1 -> Gain1/1
  Product/1 -> Gain2/1
  Psi2q/1 -> Product4/1
  Psi1d/1 -> Product3/1
  Product3/1 -> Gain3/1
  Product4/1 -> Gain4/1
  Gain2/1 -> Add3/1
  Gain1/1 -> Add3/2
  Gain/1 -> Add3/3
  Gain3/1 -> Add3/4
  Gain4/1 -> Add3/5

== system Benchmark_IEEE_standardn4/Electrical Machines/delta_cal ==
  Smd : Inport
  Delta : Integrator  InitialCondition=delta0
  Gain : Gain  Gain=wB
  delta : Outport
  wires:
  Smd/1 -> Gain/1  "Sm"
  Gain/1 -> Delta/1
  Delta/1 -> delta/1  "delta"

== matlab function Benchmark_IEEE_standardn4/NW Power/Active Power flow1 ==
  data: P18 input; P50 input; V input; V50 output; theta input; Y input; V18 output
function [V50,V18]= PowerFlow(P18,P50,V,theta,Y)
% V50=complex(0,0);
% V18=complex(0,0);
On=complex(0,0);
On2=complex(0,0);
N_Bus=68;
G=real(Y);
B=imag(Y);
% for i=1:1:N_Machine
    for k=1:1:N_Bus
        i=18;
        O=(G(i,k)*cos(theta(i)-theta(k))+B(i,k)*sin(theta(i)-theta(k)));
        On=O+On;
    end
    V18=P18*On;
% end
% for i=N_Machine+1:1:N_Bus
    for k=1:1:N_Bus
        i=50;
        O=(G(i,k)*cos(theta(i)-theta(k))+B(i,k)*sin(theta(i)-theta(k)));
        On2=O+On2;
    end
    V50=P50*On2;
% end

== matlab function Benchmark_IEEE_standardn4/MATLAB Function ==
  data: u input; y output
function y = fcn(u)

if (u(1)==0)
    u(1)=0.1;
    y = u;
else
y = u;
end

== matlab function Benchmark_IEEE_standardn4/NW Power/Active Power flow2 ==
  data: Vnew input; Pwr output; theta input; Y input
function Pwr  = PowerFlow(Vnew,theta,Y)
% Pwr=complex(0,0);
Pwr=zeros(68,1,'like',complex(0,0));
On=complex(0,0);
On2=complex(0,0);
N_Bus=68;
N_Machine=16;
G=real(Y);
B=imag(Y);
for i=1:1:N_Machine
    for k=1:1:N_Bus
        O=Vnew(k)*(G(i,k)*cos(theta(i)-theta(k))+B(i,k)*sin(theta(i)-theta(k)));
        On=O+On;
    end
    Pwr(i,1)=Vnew(i)*On;
end
for i=N_Machine+1:1:N_Bus
    for k=N_Machine+1:1:N_Bus
        O2=Vnew(k)*(G(i,k)*cos(theta(i)-theta(k))+B(i,k)*sin(theta(i)-theta(k)));
        On2=O2+On2;
    end
    Pwr(i,1)=-Vnew(i)*On2;
end

== matlab function Benchmark_IEEE_standardn4/Network/MATLAB Function ==
  data: u input; y output
function y = fcn(u)

y = (pinv(u))';

== matlab function Benchmark_IEEE_standardn4/NW Power/MATLAB Function ==
  data: MM input; Sp output; Pwr input
function Sp = fcn(MM,Pwr)
%#codegen

Sp = MM'*Pwr;

== matlab function Benchmark_IEEE_standardn4/NW Power/MATLAB Function1 ==
  data: V18 input; V18n output; V18cor input
function V18n = fcn(V18,V18cor)


V18n = V18.*V18cor;
